simulink model "Vending_model"  (R2020a)
settings: Solver=VariableStepAuto  StartTime=0.0  StopTime=10.0  RelTol=1e-3
settings Model: Creator=kiran  LastModifiedBy=kiran

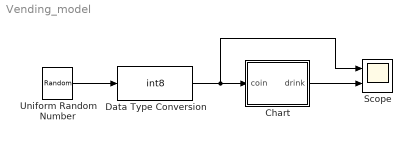
== system Vending_model ==
  Chart : Stateflow chart  TreatAsAtomicUnit=on
  Data Type Conversion : DataTypeConversion  OutDataTypeStr=int8  RndMeth=Nearest  SaturateOnIntegerOverflow=on
  Scope : Scope  NumInputPorts=2
  Uniform Random Number : UniformRandomNumber  Minimum=0  Maximum=2  Seed=337  SampleTime=10
  wires:
  Uniform Random Number/1 -> Data Type Conversion/1
  Data Type Conversion/1 -> Scope/1, Chart/1(coin)
  Chart/1(drink) -> Scope/2

== stateflow chart Vending_model/Chart ==
  state got_5
  state got_0
  state got_10
  state got_15
  state got_20
  got_15 -> got_0 [order 2] : [coin==2]{drink=1}
  (default) -> got_0
  got_0 -> got_5 [order 1] : [coin==1]{drink=0}
  got_5 -> got_10 [order 1] : [coin==1]{drink=0}
  got_20 -> got_0 [order 1] : [coin==1]{drink=1}
  got_20 -> got_5 [order 2] : [coin==2]{drink=1}
  got_0 -> got_10 [order 2] : [coin==2]{drink=0}
  got_5 -> got_15 [order 2] : [coin==2]{drink=0}
  got_10 -> got_15 [order 1] : [coin==1]{drink=0}
  got_10 -> got_20 [order 2] : [coin==2]{drink=0}
  got_15 -> got_20 [order 1] : [coin==1]{drink=0}
  data: coin input; drink output
